simulink model "condenser_test"  (R2019a)
settings: Solver=VariableStepAuto  StartTime=0.0  StopTime=100  RelTol=1e-3
settings Model: Creator=Adam  LastModifiedBy=Adam

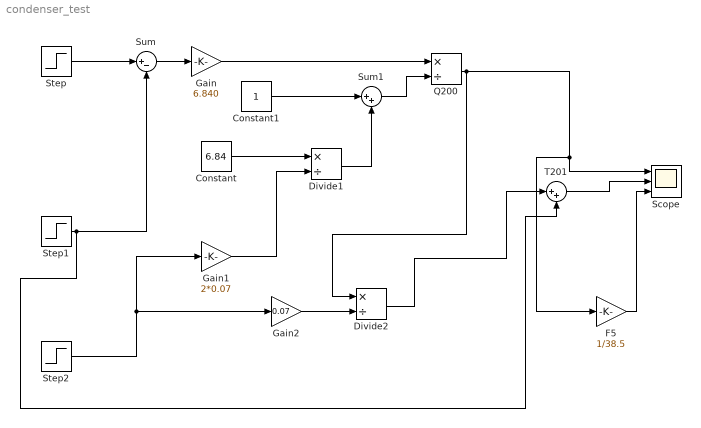
== system condenser_test ==
  Constant : Constant  Value=6.84
  Constant1 : Constant
  Divide1 : Product  Inputs=*/
  Divide2 : Product  Inputs=*/
  F5 : Gain  Gain=1/38.5
  Gain : Gain  Gain=6.840
  Gain1 : Gain  Gain=2*0.07
  Gain2 : Gain  Gain=0.07
  Q200 : Product  Inputs=*/
  Scope : Scope  NumInputPorts=3
  Step : Step  Before=0.1  SampleTime=0
  Step1 : Step  Before=0.1  SampleTime=0
  Step2 : Step  Before=0.1  SampleTime=0
  Sum : Sum  Inputs=|+-
  Sum1 : Sum  Inputs=|++
  T201 : Sum  Inputs=|++
  wires:
  Step1/1 -> Sum/2, T201/2
  Step/1 -> Sum/1
  Sum/1 -> Gain/1
  Gain/1 -> Q200/1
  Step2/1 -> Gain2/1, Gain1/1
  Constant/1 -> Divide1/1
  Gain1/1 -> Divide1/2
  Sum1/1 -> Q200/2
  Constant1/1 -> Sum1/1
  Divide1/1 -> Sum1/2
  Q200/1 -> Divide2/1, Scope/1, F5/1
  Gain2/1 -> Divide2/2
  Divide2/1 -> T201/1
  T201/1 -> Scope/2
  F5/1 -> Scope/3
